simulink model "Loop_model"  (R2023b)
settings: Solver=ode5  StartTime=0.0  StopTime=1e4  RelTol=1e-3
values from neighbouring files (symbols this model uses):
  a = 6.851221970532768e+03    (= 6851.22197053)    [complete_model.m]
  alpha1 = 0.4    [complete_model.m]
  alpha2 = 0.1    [complete_model.m]
  alpha3 = 0.5    [complete_model.m]
  bias_mag = [0.581454665479 0.362156984222 0.728527824295]    [bias_bad.mat]    (also in complete_model.m = bias_mag./norm(bias_mag))
  D = zeros(3)    [complete_model.m]
  e = 0    [complete_model.m]
  FOV_earth = deg2rad(33)    [complete_model.m]
  freq_acds = 30    [complete_model.m]
  freq_earth = 30    [complete_model.m]
  freq_mag = 30    [complete_model.m]
  freq_sun = 30    [complete_model.m]
  I = diag([I1 I2 I3])    [complete_model.m]    (also in compute_integral.m = I + (y(i + 1) + y(i) ) * (t(i + 1) - t(i)) * 0.5)
  Iinv = I\eye(3)    [complete_model.m]
  jb = [0.01; 0.05; 0.01]    [complete_model.m]
  k_gain = (4*pi/T) * (1 + sin(chsi)) * I2    [complete_model.m]
  mu = astroConstants(13)    [complete_model.m]
  n = sqrt(mu/a^3)    [complete_model.m]
  noise_sd_mag = 1.18*1e-12    (= 1.18e-12)    [complete_model.m]
  omega0 = 0.06 * rand(3,1)    [complete_model.m]
  omegaE = deg2rad(15)/3600    [complete_model.m]
  rs = -rr    [complete_model.m]
  s0 = 2*pi*rand(3,1)    [complete_model.m]
  tol = 0.2    [complete_model.m]
undefined symbols (not defined in the file or in its folder): flag_h, gh, magnitude, s_h, s_m, s_s, v_h, v_m, v_s
libraries: vrlib x9, matrix_library x6, cstextras x3, simulink x3, simulink_extras x1
(part 3 of 3)

== system Loop_model/Kinematics/Kinematics 313/s_313 - A/R3_1 ==
  x : Inport
  Constant : Constant  Value=[0; 0; 1]
  Constant1 : Constant  Value=0
  Cos : Trigonometry  Operator=cos
  Gain : Gain  Gain=-1
  Matrix Concatenate : Concatenate  NumInputs=3  Mode=Multidimensional array  ConcatenateDimension=2
  Sin : Trigonometry
  Vector Concatenate : Concatenate  NumInputs=3
  Vector Concatenate1 : Concatenate  NumInputs=3
  R3 : Outport
  wires:
  Matrix Concatenate/1 -> R3/1
  Constant1/1 -> Vector Concatenate1/3, Vector Concatenate/3
  x/1 -> Cos/1, Sin/1
  Vector Concatenate1/1 -> Matrix Concatenate/2
  Gain/1 -> Vector Concatenate/2
  Constant/1 -> Matrix Concatenate/3
  Cos/1 -> Vector Concatenate/1, Vector Concatenate1/2
  Sin/1 -> Gain/1, Vector Concatenate1/1
  Vector Concatenate/1 -> Matrix Concatenate/1

== system Loop_model/Kinematics/Kinematics 313/s_313 - A/R3_2 ==
  x : Inport
  Constant : Constant  Value=[0; 0; 1]
  Constant1 : Constant  Value=0
  Cos : Trigonometry  Operator=cos
  Gain : Gain  Gain=-1
  Matrix Concatenate : Concatenate  NumInputs=3  Mode=Multidimensional array  ConcatenateDimension=2
  Sin : Trigonometry
  Vector Concatenate : Concatenate  NumInputs=3
  Vector Concatenate1 : Concatenate  NumInputs=3
  R3 : Outport
  wires:
  Vector Concatenate/1 -> Matrix Concatenate/1
  Sin/1 -> Vector Concatenate1/1, Gain/1
  Cos/1 -> Vector Concatenate1/2, Vector Concatenate/1
  Constant/1 -> Matrix Concatenate/3
  Gain/1 -> Vector Concatenate/2
  Vector Concatenate1/1 -> Matrix Concatenate/2
  x/1 -> Sin/1, Cos/1
  Constant1/1 -> Vector Concatenate/3, Vector Concatenate1/3
  Matrix Concatenate/1 -> R3/1

== system Loop_model/Control/Slew Maneuver/Control Logic/Subsystem/Assembly Matrix ==
  Bm : Inport
  Constant : Constant  Value=0
  Constant1 : Constant
  Constant2 : Constant  Value=0
  Demux : Demux  Outputs=3
  Gain : Gain  Gain=-1
  Gain1 : Gain  Gain=-1
  Gain2 : Gain  Gain=-1
  Matrix Concatenate : Concatenate  NumInputs=3  Mode=Multidimensional array  ConcatenateDimension=2
  Vector Concatenate : Concatenate  NumInputs=3
  Vector Concatenate1 : Concatenate  NumInputs=3
  Vector Concatenate2 : Concatenate  NumInputs=3
  Matrix : Outport
  wires:
  Constant/1 -> Vector Concatenate/1
  Bm/1 -> Demux/1
  Gain/1 -> Vector Concatenate/2
  Demux/3 -> Vector Concatenate1/1, Gain/1
  Demux/2 -> Gain2/1, Vector Concatenate/3
  Constant1/1 -> Vector Concatenate1/2
  Gain1/1 -> Vector Concatenate1/3
  Demux/1 -> Vector Concatenate2/2, Gain1/1
  Gain2/1 -> Vector Concatenate2/1
  Constant2/1 -> Vector Concatenate2/3
  Vector Concatenate1/1 -> Matrix Concatenate/2
  Vector Concatenate/1 -> Matrix Concatenate/1
  Vector Concatenate2/1 -> Matrix Concatenate/3
  Matrix Concatenate/1 -> Matrix/1

== system Loop_model/Control/Slew Maneuver/Control Logic/Subsystem1/Assembly Matrix ==
  B_m : Inport
  Constant : Constant  Value=0
  Constant1 : Constant
  Demux : Demux  Outputs=3
  Gain : Gain  Gain=-1
  Gain1 : Gain  Gain=-1
  Gain2 : Gain  Gain=-1
  Matrix Concatenate : Concatenate  NumInputs=3  Mode=Multidimensional array  ConcatenateDimension=2
  Vector Concatenate : Concatenate  NumInputs=3
  Vector Concatenate1 : Concatenate  NumInputs=3
  Vector Concatenate2 : Concatenate  NumInputs=3
  "Matrix " : Outport
  wires:
  B_m/1 -> Demux/1
  Constant1/1 -> Vector Concatenate/1
  Gain/1 -> Vector Concatenate/2
  Demux/3 -> Gain/1, Vector Concatenate1/1
  Demux/2 -> Gain2/1, Vector Concatenate/3
  Gain1/1 -> Vector Concatenate1/3
  Demux/1 -> Gain1/1, Vector Concatenate2/2
  Constant/1 -> Vector Concatenate1/2, Vector Concatenate2/3
  Gain2/1 -> Vector Concatenate2/1
  Vector Concatenate1/1 -> Matrix Concatenate/2
  Vector Concatenate/1 -> Matrix Concatenate/1
  Vector Concatenate2/1 -> Matrix Concatenate/3
  Matrix Concatenate/1 -> "Matrix "/1

== system Loop_model/Control/Slew Maneuver/compute alphadots/Invert/Determinant of 3x3 Matrix ==
  Matrix : Inport  PortDimensions=[3 3]
  Product{,1..5} (6 alike) : Product  Inputs=1  SaturateOnIntegerOverflow=on  OutDataTypeStr=Inherit: Same as first input
  Reshape : Reshape  OutputDimensionality=Column vector (2-D)
  Sum : Sum  Inputs=+--++-  SaturateOnIntegerOverflow=on
  a(1,1),a(2,2),a(3,3) : Selector  InputPortWidth=9  IndexOptions=Index vector (dialog)  Indices=[1 5 9]  OutputSizes=1
  a(1,1),a(2,3),a(3,2) : Selector  InputPortWidth=9  IndexOptions=Index vector (dialog)  Indices=[1 6 8]  OutputSizes=1
  a(1,2),a(2,1),a(3,3) : Selector  InputPortWidth=9  IndexOptions=Index vector (dialog)  Indices=[2 4 9]  OutputSizes=1
  a(1,2),a(2,3),a(3,1) : Selector  InputPortWidth=9  IndexOptions=Index vector (dialog)  Indices=[3 4 8]  OutputSizes=1
  a(1,3),a(2,1),a(3,2) : Selector  InputPortWidth=9  IndexOptions=Index vector (dialog)  Indices=[2 6 7]  OutputSizes=1
  a(1,3),a(2,2),a(3,1) : Selector  InputPortWidth=9  IndexOptions=Index vector (dialog)  Indices=[3 5 7]  OutputSizes=1
  det : Outport  PortDimensions=1  VectorParamsAs1DForOutWhenUnconnected=off
  wires:
  Reshape/1 -> a(1,1),a(2,3),a(3,2)/1, a(1,1),a(2,2),a(3,3)/1, a(1,3),a(2,2),a(3,1)/1, a(1,3),a(2,1),a(3,2)/1, a(1,2),a(2,3),a(3,1)/1, a(1,2),a(2,1),a(3,3)/1
  Sum/1 -> det/1  "det(Matrix)"
  Matrix/1 -> Reshape/1
  Product5/1 -> Sum/6
  Product4/1 -> Sum/5
  Product3/1 -> Sum/4
  Product2/1 -> Sum/3
  Product1/1 -> Sum/2
  Product/1 -> Sum/1
  a(1,3),a(2,2),a(3,1)/1 -> Product5/1
  a(1,3),a(2,1),a(3,2)/1 -> Product4/1
  a(1,2),a(2,3),a(3,1)/1 -> Product3/1
  a(1,2),a(2,1),a(3,3)/1 -> Product2/1
  a(1,1),a(2,3),a(3,2)/1 -> Product1/1
  a(1,1),a(2,2),a(3,3)/1 -> Product/1

== matlab function Loop_model/Environment/Magnetic Field/MATLAB Function ==
  data: r input; B output; theta input; phi input; gh input
function B = calculateField(r, theta, phi, gh)

N = 13;         % Order of the field
lat = pi/2 - theta;
lon = phi;

R = 6371.2;     % Radius of Earth in IGRF
ratio = R / r;

sin_lat = sin(lat);
cos_lat = cos(lat);
sin_lon = sin(lon);
cos_lon = cos(lon);

npq = (N * (N+3)) / 2;

p = zeros(npq, 1);
p(1) = 2*sin_lat;
p(2) = 2*cos_lat;
p(3) = 4.5*sin_lat^2 - 1.5;
p(4) = 3*sqrt(3) * cos_lat * sin_lat;

q = zeros(npq, 1);
q(1) = -cos_lat;
q(2) = sin_lat;
q(3) = -3 * cos_lat * sin_lat;
q(4) = sqrt(3) * (sin_lat^2 - cos_lat^2);

sl = zeros(N+1, 1);
sl(1) = sin_lon;

cl = zeros(N+1, 1);
cl(1) = cos_lon;

Bx = 0; By = 0; Bz = 0;
l = 1; n = 0; m = 1;
fn = nan; rr = nan;

for k = 1:npq

    if n < m
        m = 0;
        n = n + 1;
        rr = ratio^(n+2);
        fn = n;
    end

    fm = m;

    if k >= 5

        if m == n
            a = sqrt(1 - 0.5/fm);
            j = k - n - 1;
            p(k) = (1 + 1/fm) * a * cos_lat * p(j);
            q(k) = a * (cos_lat * q(j) + sin_lat/fm * p(j));
            sl(m) = sl(m-1)*cl(1) + cl(m-1)*sl(1);
            cl(m) = cl(m-1)*cl(1) - sl(m-1)*sl(1);
        else
            a = sqrt(fn^2 - fm^2);
            b = sqrt((fn-1)^2 - fm^2) / a;
            c = (2*fn - 1) / a;
            ii = k - n;
            j = k - 2*n + 1;
            p(k) = (fn+1) * (c * sin_lat/fn * p(ii) - b/(fn-1) * p(j));
            q(k) = c * (sin_lat * q(ii) - cos_lat/fn * p(ii)) - b * q(j);
        end

    end

    a = rr * gh(l);
    
    if m == 0

        Bx = Bx + a*q(k);
        Bz = Bz - a*p(k);
        
        l = l + 1;

    else
        
        b = rr * gh(l+1);
        c = a*cl(m) + b*sl(m);
        Bx = Bx + c * q(k);
        Bz = Bz - c * p(k);
        
        if cos_lat > 0
            By = By + (a*sl(m) - b*cl(m)) * fm * p(k)/((fn+1) * cos_lat);
        else
            By = By + (a*sl(m) - b*cl(m)) * q(k) * sin_lat;
        end
        
        l = l + 2;

    end

    m = m + 1;

end

B_NED = [Bx; By; Bz] * 1e-9;

% Convert NED to ECEF
R = [-sin_lat * cos_lon,    -sin_lon,   -cos_lat * cos_lon;
     -sin_lat * sin_lon,    cos_lon,    -cos_lat * sin_lon;
     cos_lat,               0,          -sin_lat            ];

B = R * B_NED;

== matlab function Loop_model/Control/Slew Maneuver/Control Logic/Subsystem/MATLAB Function ==
  data: A input; x output; b input
function x = solve(A, b)

x = A \ b;

== matlab function Loop_model/Attitude Determination/Statistical Method/MATLAB Function ==
  data: A input; U output; V output
function [U,V] = SVD(A)

[U,~,V] = svd(A);

end

== matlab function Loop_model/Control/Slew Maneuver/Control Logic/Subsystem1/MATLAB Function ==
  data: A input; x output; b input
function x = solve(A, b)

x = A \ b;
